simulink model "EEMotor_Build"  (R2026a)
settings: Solver=VariableStepAuto
libraries: nesl_utility x5, sm_lib x1
settings Model: Creator=eqtran103  LastModifiedBy=eqtran103

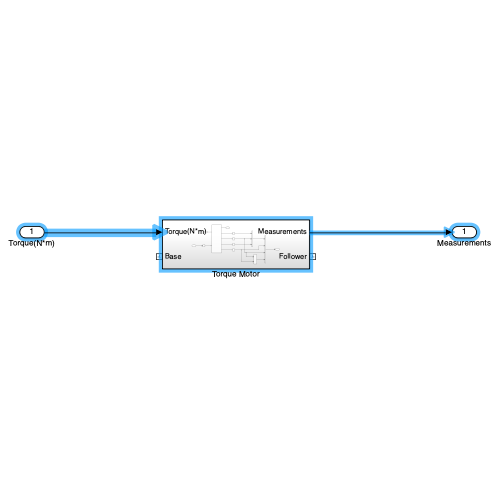
[thumbnail: Simulink's stored preview of the top-level diagram]
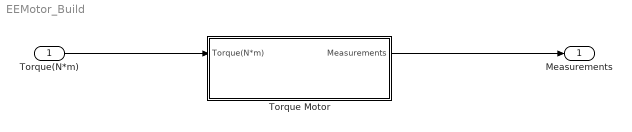
== system EEMotor_Build ==
  Torque(N*m) : Inport
  Torque Motor : Subsystem
  Measurements : Outport
  wires:
  Torque(N*m)/1 -> Torque Motor/1(Torque(N*m))
  Torque Motor/1(Measurements) -> Measurements/1

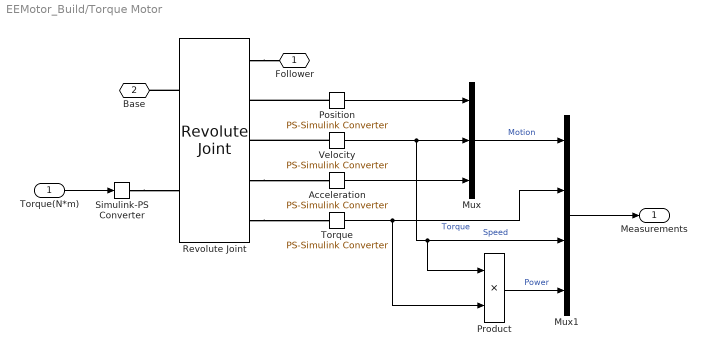
== system EEMotor_Build/Torque Motor ==
  Torque(N*m) : Inport
  Acceleration : nesl_utility/PS-Simulink Converter  PhysicalDomain=network_engine_domain  SubClassName=ps_output  LeftPortType=input  RightPortType=output  PseudoPeriodic=off  Frequencies=[]  VectorFormat=inherit  Unit=inherit  AffineConversion=off
  Mux : Mux  Inputs=3
  Mux1 : Mux
  Position : nesl_utility/PS-Simulink Converter  PhysicalDomain=network_engine_domain  SubClassName=ps_output  LeftPortType=input  RightPortType=output  PseudoPeriodic=off  Frequencies=[]  VectorFormat=inherit  Unit=inherit  AffineConversion=off
  Product : Product
  Revolute Joint : sm_lib/Joints/Revolute Joint  JointMode=Normal  CompositeWrenchDir=FollowerOnBase  CompositeWrenchFrame=BaseFrame  SenseConstraintForce=off  SenseConstraintTorque=off  SenseTotalForce=off  SenseTotalTorque=off  PositionTargetSpecify=off  PositionTargetPriority=High  PositionTargetValue=0  PositionTargetValueUnits=deg  VelocityTargetSpecify=off  VelocityTargetPriority=High  VelocityTargetValue=0  VelocityTargetValueUnits=deg/s  EquilibriumPosition=0  EquilibriumPositionUnits=deg  SpringStiffness=0  SpringStiffnessUnits=N*m/deg  DampingCoefficient=0  DampingCoefficientUnits=N*m/(deg/s)  LowerLimitSpecify=off  LowerLimitBound=-90  LowerLimitBoundUnits=deg  LowerLimitStiffness=1e4  LowerLimitStiffnessUnits=N*m/deg  LowerLimitDamping=10  LowerLimitDampingUnits=N*m/(deg/s)  LowerLimitTransitionRegionWidth=0.1  LowerLimitTransitionRegionWidthUnits=deg  UpperLimitSpecify=off  UpperLimitBound=90  UpperLimitBoundUnits=deg  UpperLimitStiffness=1e4  UpperLimitStiffnessUnits=N*m/deg  UpperLimitDamping=10  UpperLimitDampingUnits=N*m/(deg/s)  UpperLimitTransitionRegionWidth=0.1  UpperLimitTransitionRegionWidthUnits=deg  TorqueActuationMode=InputTorque  MotionActuationMode=ComputedMotion  SensePosition=on  SenseVelocity=on  SenseAcceleration=on  SenseTorqueForce=on  SenseLowerLimitTorqueForce=off  SenseUpperLimitTorqueForce=off
  Simulink-PS Converter : nesl_utility/Simulink-PS Converter  PhysicalDomain=network_engine_domain  SubClassName=ps_input  LeftPortType=input  RightPortType=output  PseudoPeriodic=off  Frequencies=[]  NoiseDistribution=none  NoiseParameters=[]  Unit=1  AffineConversion=off  FilteringAndDerivatives=provide  SimscapeFilterOrder=1  InputFilterTimeConstant=0.001  UdotUserProvided=0
  Torque : nesl_utility/PS-Simulink Converter  PhysicalDomain=network_engine_domain  SubClassName=ps_output  LeftPortType=input  RightPortType=output  PseudoPeriodic=off  Frequencies=[]  VectorFormat=inherit  Unit=inherit  AffineConversion=off
  Velocity : nesl_utility/PS-Simulink Converter  PhysicalDomain=network_engine_domain  SubClassName=ps_output  LeftPortType=input  RightPortType=output  PseudoPeriodic=off  Frequencies=[]  VectorFormat=inherit  Unit=inherit  AffineConversion=off
  Follower : PMIOPort  Side=Right
  Base : PMIOPort  Port=2  Side=Left
  Measurements : Outport
  wires:
  Product/1 -> Mux1/4  "Power"
  Position/1 -> Mux/1
  Torque(N*m)/1 -> Simulink-PS Converter/1
  Torque/1 -> Product/2, Mux1/2  "Torque"
  Mux/1 -> Mux1/1  "Motion"
  Acceleration/1 -> Mux/3
  Velocity/1 -> Product/1, Mux1/3, Mux/2  "Speed"
  Mux1/1 -> Measurements/1
  connections:
  Revolute Joint/LConn1 -- Base/RConn1
  Revolute Joint/RConn1 -- Follower/RConn1
  Position/LConn1 -- Revolute Joint/RConn2
  Velocity/LConn1 -- Revolute Joint/RConn3
  Revolute Joint/RConn4 -- Acceleration/LConn1
  Simulink-PS Converter/RConn1 -- Revolute Joint/LConn2
  Revolute Joint/RConn5 -- Torque/LConn1
